simulink model "FullModel"  (R2023a)
settings: Solver=ode23t  StartTime=0.0  StopTime=10  RelTol=1e-3
values from neighbouring files (symbols this model uses):
  XMAX = 5    [PrintFasePortret.m]
libraries: simulink x2
settings Model: SimulationMode=accelerator  Creator=KozlovM  LastModifiedBy=Алексей

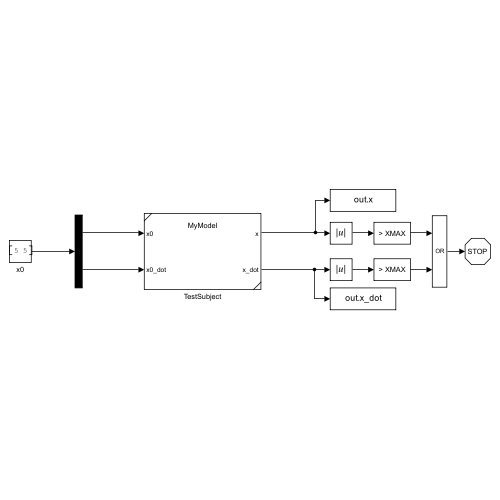
[thumbnail: Simulink's stored preview of the top-level diagram]
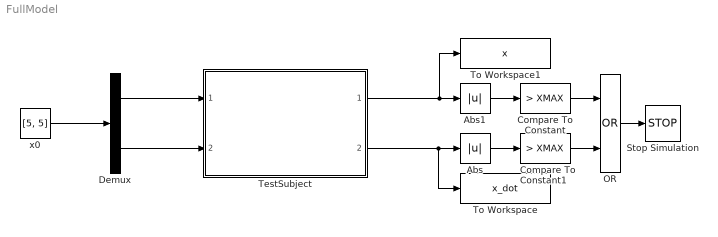
== system FullModel ==
  Abs : Abs  SaturateOnIntegerOverflow=off
  Abs1 : Abs  SaturateOnIntegerOverflow=off
  Compare To Constant : simulink/Logic and Bit Operations/Compare To Constant  relop=>  const=XMAX  OutDataTypeStr=boolean
  Compare To Constant1 : simulink/Logic and Bit Operations/Compare To Constant  relop=>  const=XMAX  OutDataTypeStr=boolean
  Demux : Demux  Outputs=2
  OR : Logic  Operator=OR  AllPortsSameDT=off  OutDataTypeStr=boolean
  Stop Simulation : Stop
  TestSubject : Subsystem  ReferencedSubsystem=MyModel
  To Workspace : ToWorkspace  VariableName=x_dot  SampleTime=-1
  To Workspace1 : ToWorkspace  VariableName=x  SampleTime=-1
  x0 : Constant  Value=[5, 5]  VectorParams1D=off
  wires:
  Abs1/1 -> Compare To Constant/1
  Abs/1 -> Compare To Constant1/1
  OR/1 -> Stop Simulation/1
  Compare To Constant/1 -> OR/1
  Compare To Constant1/1 -> OR/2
  TestSubject/1 -> To Workspace1/1, Abs1/1
  TestSubject/2 -> To Workspace/1, Abs/1
  Demux/2 -> TestSubject/2
  Demux/1 -> TestSubject/1
  x0/1 -> Demux/1
